simulink model "Fuzzy_Control_Pendulum_Cau_2"  (Simulink 7.4)
settings: Solver=ode5  StartTime=0.0  StopTime=60  FixedStep=0.001  RelTol=1e-3
libraries: fuzblock x1
settings Model: Creator=lemin  LastModifiedBy=lemin

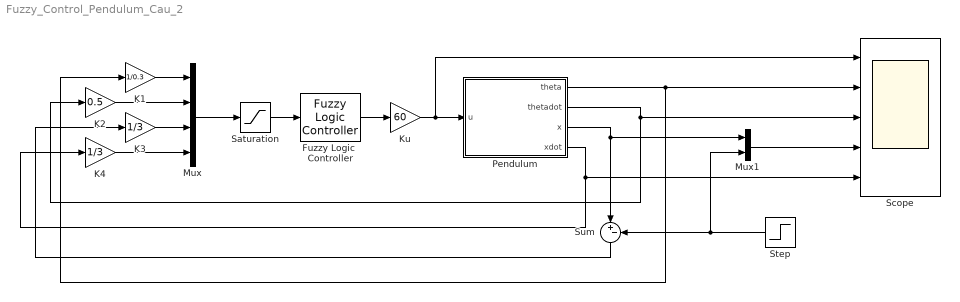
== system Fuzzy_Control_Pendulum_Cau_2 ==
  Fuzzy Logic  Controller : fuzblock/Fuzzy Logic  Controller  SystemSampleTime=-1  fis='Pendulum.fis'
  K1 : Gain  Gain=1/0.3  ParameterDataType=fixdt(1, 16)  ParameterScaling=2^0  OutDataType=fixdt(1, 16)  OutScaling=2^0
  K2 : Gain  Gain=0.5  ParameterDataType=fixdt(1, 16)  ParameterScaling=2^0  OutDataType=fixdt(1, 16)  OutScaling=2^0
  K3 : Gain  Gain=1/3  ParameterDataType=fixdt(1, 16)  ParameterScaling=2^0  OutDataType=fixdt(1, 16)  OutScaling=2^0
  K4 : Gain  Gain=1/3  ParameterDataType=fixdt(1, 16)  ParameterScaling=2^0  OutDataType=fixdt(1, 16)  OutScaling=2^0
  Ku : Gain  Gain=60  ParameterDataType=fixdt(1, 16)  ParameterScaling=2^0  OutDataType=fixdt(1, 16)  OutScaling=2^0
  Mux : Mux
  Mux1 : Mux  Inputs=2
  Pendulum : Subsystem  mask{p=0.5, m=0.3, l=1, g=9.81, thetadot0=-0.1, thetadot1=-0.2, xdot0=-0.1, xdot1=0.2}
      mask prompts: p "Khoi luong xe"; m "Khoi luong con lac"; l "Chieu dai day"; g "Gia toc trong truong"; thetadot0 "Initial theta"; thetadot1 "Initial thetadot"; xdot0 "Initial x"; xdot1 "Initial xdot"
  Saturation : Saturate  UpperLimit=1  LowerLimit=-1  OutDataType=fixdt(1, 16)  OutScaling=2^0
  Scope : Scope  NumInputPorts=5
      settings: TimeRange=60  YMin=13.3~-90~-12~0~50  YMax=13.85~0~0~2750~275
  Step : Step  Time=20  SampleTime=0.001
  Sum : Sum  Inputs=|+-  OutDataType=fixdt(1, 16)  OutScaling=2^0
  wires:
  Fuzzy Logic  Controller/1 -> Ku/1
  Ku/1 -> Pendulum/1(u), Scope/1
  Saturation/1 -> Fuzzy Logic  Controller/1
  Mux/1 -> Saturation/1
  Pendulum/2(thetadot) -> K2/1, Scope/3
  Pendulum/4(xdot) -> K4/1, Scope/5
  K1/1 -> Mux/1
  K2/1 -> Mux/2
  K3/1 -> Mux/3
  K4/1 -> Mux/4
  Pendulum/3(x) -> Sum/1, Mux1/1
  Step/1 -> Sum/2, Mux1/2
  Sum/1 -> K3/1
  Pendulum/1(theta) -> Scope/2, K1/1
  Mux1/1 -> Scope/4

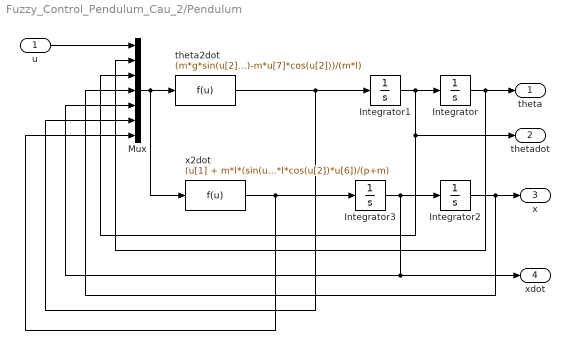
== system Fuzzy_Control_Pendulum_Cau_2/Pendulum ==
  u : Inport  OutDataType=fixdt(1, 16)  OutScaling=2^0
  Integrator : Integrator  InitialCondition=thetadot0
  Integrator1 : Integrator  InitialCondition=thetadot1
  Integrator2 : Integrator  InitialCondition=xdot0
  Integrator3 : Integrator  InitialCondition=xdot1
  Mux : Mux  Inputs=7
  theta2dot : Fcn  Expr=(m*g*sin(u[2])-m*u[7]*cos(u[2]))/(m*l)
  x2dot : Fcn  Expr=(u[1] + m*l*(sin(u[2]))*(u[3])^2 - m*l*cos(u[2])*u[6])/(p+m)
  theta : Outport  OutDataType=fixdt(1, 16)  OutScaling=2^0
  thetadot : Outport  Port=2  OutDataType=fixdt(1, 16)  OutScaling=2^0
  x : Outport  Port=3  OutDataType=fixdt(1, 16)  OutScaling=2^0
  xdot : Outport  Port=4  OutDataType=fixdt(1, 16)  OutScaling=2^0
  wires:
  u/1 -> Mux/1
  Mux/1 -> theta2dot/1, x2dot/1
  theta2dot/1 -> Integrator1/1, Mux/6
  Integrator1/1 -> Integrator/1, thetadot/1, Mux/3
  Integrator/1 -> theta/1, Mux/2
  x2dot/1 -> Integrator3/1, Mux/7
  Integrator3/1 -> Integrator2/1, Mux/5, xdot/1
  Integrator2/1 -> Mux/4, x/1
